simulink model "verify_Pressure_Drop_staticHeight_mdl"  (R2016b)
settings: Solver=VariableStepDiscrete  StartTime=0.0  StopTime=10  MaxStep=1  RelTol=1e-3  EnableMultiTasking=on
libraries: carnot x2
settings Model: Creator=drhf  LastModifiedBy=srrt
settings DataIOCC: LimitDataPoints=on  SaveFormat=Array  SignalLoggingSaveFormat=ModelDataLogs
settings OptimizationCC: ExpressionDepthLimit=2147483647  LifeSpan=inf
settings DebuggingCC: UnderspecifiedInitializationDetection=Classic  MergeDetectMultiDrivingBlocksExec=none  SolverPrmCheckMsg=warning  FcnCallInpInsideContextMsg=warning  StateNameClashWarn=warning  SFUnexpectedBacktrackingDiag=warning  SFNoUnconditionalDefaultTransitionDiag=warning  SFExecutionAtInitializationDiag=none
settings HardwareCC: ProdBitPerPointer=32  ProdBitPerSizeT=32  ProdBitPerPtrDiffT=32  ProdLargestAtomicFloat=None  ProdIntDivRoundTo=Undefined  ProdEndianess=Unspecified  ProdWordSize=32  ProdHWDeviceType=32-bit Generic
settings ModelReferenceCC: PropagateSignalLabelsOutOfModel=off
settings GRTTargetCC: TargetLangStandard=C89/C90 (ANSI)  GeneratePreprocessorConditionals=Disable all  CombineOutputUpdateFcns=off  GRTInterface=on
settings ConfigComp: CovMetricSettings=dw  CovHtmlReporting=on  CovSaveCumulativeToWorkspaceVar=on  CovSaveSingleToWorkspaceVar=on  CovExternalEMLEnable=off

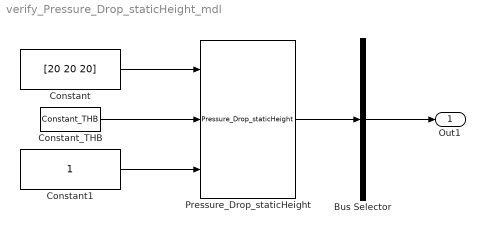
== system verify_Pressure_Drop_staticHeight_mdl ==
  Bus Selector : BusSelector  OutputSignals=Pressure,DPConstant,DPLinear,DPQuadratic  OutputAsBus=on
  Constant : Constant  Value=[20 20 20]
  Constant1 : Constant
  Constant_THB : carnot/Source/Simple/Constant_THB  t=40  mdot=100/3600  p=1e5  mID=Full Pressure Drop with Static Height  fluid=Water  mix=0  mix2=0  mix3=0  dia=1  hgt=0
  Pressure_Drop_staticHeight : carnot/Basic/Pressure_Drop/Pressure_Drop_staticHeight
  Out1 : Outport
  wires:
  Constant_THB/1 -> Pressure_Drop_staticHeight/2
  Pressure_Drop_staticHeight/1 -> Bus Selector/1
  Bus Selector/1 -> Out1/1
  Constant/1 -> Pressure_Drop_staticHeight/1
  Constant1/1 -> Pressure_Drop_staticHeight/3
